simulink model "Problem5_Circuit_Simulation"  (R2020b)
settings: Solver=VariableStepAuto  StartTime=0.0  StopTime=10  RelTol=1e-3
PreLoadFcn:
  | clearvars
  | load('Data.mat')
undefined symbols (not defined in the file): C, R, sigbuilder_block
settings Model: Creator=vigne  LastModifiedBy=prabhudevmaddipudi

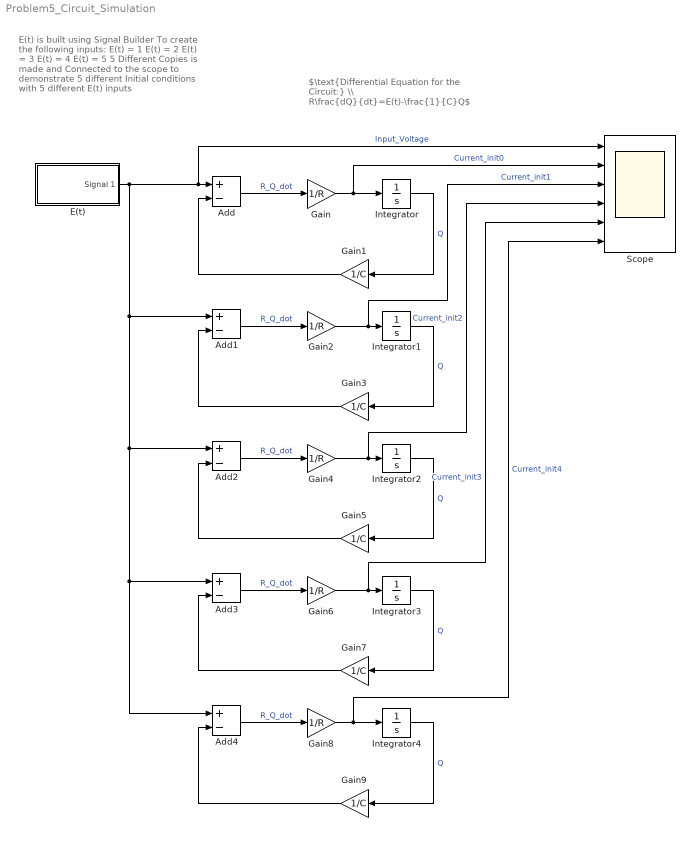
== system Problem5_Circuit_Simulation ==
  note: E(t) is built using Signal Builder
      | To create the following inputs:
      | E(t) = 1
      | E(t) = 2
      | E(t) = 3
      | E(t) = 4
      | E(t) = 5
      | 5 Different Copies is made and
      | Connected to the scope to
      | demonstrate 5 different Initial conditions
      | with 5 different E(t) inputs
  note: $\text{Differential Equation for the Circuit:} \\ R\frac{dQ}{dt}=E(t)-\frac{1}{C}Q$
  Add{,1..4} (5 alike) : Sum  Inputs=+-
  E(t) : Subsystem  Tag=STV Subsys  LoadFcn=sigbuilder_block('load');  StartFcn=sigbuilder_block('start');  StopFcn=sigbuilder_block('stop');  ClipboardFcn=sigbuilder_block('clipboard');  mask(Sigbuilder block){tuvar=[0:10]}
      mask help: Simulink:masks:SigbuilderBlock_MD
      mask init:
      | if ~strcmp(get_param(bdroot(gcbh),'SimulationStatus'),'stopped') tuvar = sigbuilder_block('maskInit'); end
      settings: CopyFcn=sigbuilder_block('copy');  DeleteFcn=sigbuilder_block('delete');  ModelCloseFcn=sigbuilder_block('modelClose');  PreSaveFcn=sigbuilder_block('preSave');  PauseFcn=sigbuilder_block('pause');  ContinueFcn=sigbuilder_block('continue');  NameChangeFcn=sigbuilder_block('namechange');  OpenFcn=sigbuilder_block('open',[437.6 153 550.4 359.25 ]);  CloseFcn=sigbuilder_block('close');
      mask Display: plot(0, 0, 100, 100,[2, 2, 32, 32, 2], [68, 8, 8, 68, 68],[32, 2], [38, 38], [32, 19, 2],[53, 60, 44], [32, 17, 17, 2],[16, 16, 31, 31]);txt = getActiveGroup(gcbh);text(2, 100, txt,'verticalAlignment', 'top');
  Gain{,2,4,6,8} (5 alike) : Gain  Gain=1/R
  Gain{1,3,5,7,9} (5 alike) : Gain  Gain=1/C
  Integrator : Integrator
  Integrator1 : Integrator  InitialCondition=1
  Integrator2 : Integrator  InitialCondition=2
  Integrator3 : Integrator  InitialCondition=3
  Integrator4 : Integrator  InitialCondition=4
  Scope : Scope  NumInputPorts=6
  wires:
  Add/1 -> Gain/1  "R_Q_dot"
  Gain/1 -> Scope/2, Integrator/1  "Current_init0"
  Integrator/1 -> Gain1/1  "Q"
  Gain1/1 -> Add/2
  Gain3/1 -> Add1/2
  Gain2/1 -> Scope/3, Integrator1/1  "Current_init1"
  Integrator1/1 -> Gain3/1  "Q"
  Add1/1 -> Gain2/1  "R_Q_dot"
  Gain5/1 -> Add2/2
  Gain4/1 -> Scope/4, Integrator2/1  "Current_init2"
  Integrator2/1 -> Gain5/1  "Q"
  Add2/1 -> Gain4/1  "R_Q_dot"
  Gain7/1 -> Add3/2
  Gain6/1 -> Scope/5, Integrator3/1  "Current_init3"
  Integrator3/1 -> Gain7/1  "Q"
  Add3/1 -> Gain6/1  "R_Q_dot"
  Gain9/1 -> Add4/2
  Gain8/1 -> Scope/6, Integrator4/1  "Current_init4"
  E(t)/1(Signal 1) -> Add2/1, Add3/1, Add4/1, Add1/1, Scope/1, Add/1  "Input_Voltage"
  Integrator4/1 -> Gain9/1  "Q"
  Add4/1 -> Gain8/1  "R_Q_dot"

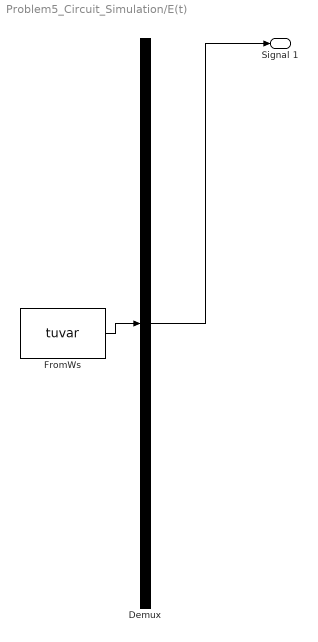
== system Problem5_Circuit_Simulation/E(t) ==
  Demux : Demux  Tag=STV Demux  Outputs=1
      settings: DisplayOption=none
  FromWs : FromWorkspace  Tag=STV FromWs  VariableName=tuvar  OutputAfterFinalValue=Setting to zero
      SigBuilderData=|
      | common.afterFinalStr = 'Set to zero'
      | common.sampleTime = '0'
      | dataSet.timeRange = [0 10]
      | dataSet.name = 'Group 1'
      | sbobj.Groups.Name = 'Group 1'
      | sbobj.Groups.Signals.Name = 'Signal 1'
      | sbobj.Groups.Signals.XData = [0 1 1 2 2 3 3 4 4 5 5 6 6 7 7 8 8 9 9 10]
      | sbobj.Groups.Signals.YData = [0 0 1 1 0 0 2 2 0 0 3 3 0 0 4 4 0 0 5 5]
  Signal 1 : Outport  Tag=STV Outport
  wires:
  Demux/1 -> Signal 1/1
  FromWs/1 -> Demux/1
